simulink model "sampleModel344"  (R2021b)
settings: Solver=VariableStepAuto  StartTime=0.0  StopTime=10.0  RelTol=1e-3
undefined symbols (not defined in the file or in its folder): DiscIntNeverNeededParam
libraries: simulink x1
settings Model: Creator=user  LastModifiedBy=user

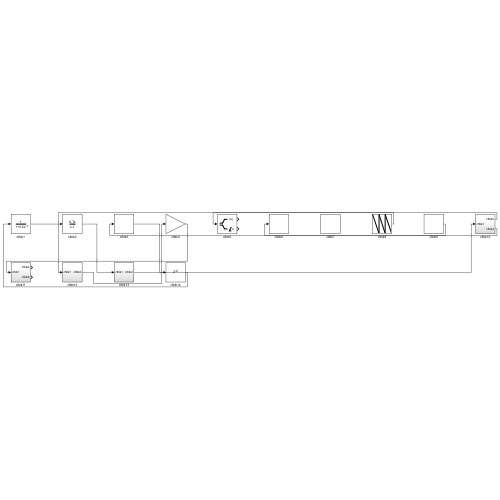
[thumbnail: Simulink's stored preview of the top-level diagram]
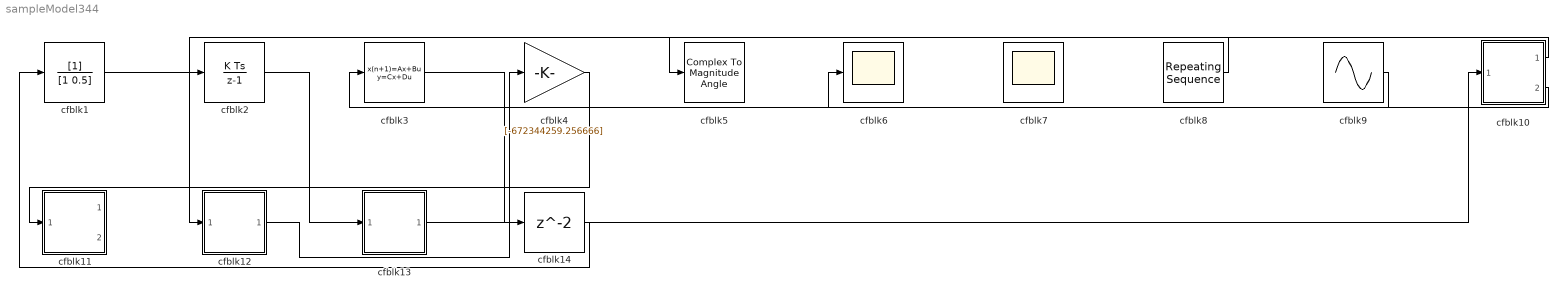
== system sampleModel344 ==
  cfblk1 : DiscreteFilter  SampleTime=1
  cfblk10 : Subsystem
  cfblk11 : Subsystem
  cfblk12 : Subsystem
  cfblk13 : Subsystem
  cfblk14 : Delay  SampleTime=1
  cfblk2 : DiscreteIntegrator  ICPrevOutput=DiscIntNeverNeededParam  ICPrevScaledInput=DiscIntNeverNeededParam
  cfblk3 : DiscreteStateSpace
  cfblk4 : Gain  Gain=[-672344259.256666]
  cfblk5 : ComplexToMagnitudeAngle
  cfblk6 : Scope
  cfblk7 : Scope
      settings: Floating=on
  cfblk8 : simulink/Sources/Repeating Sequence  rep_seq_t=[0 2]  rep_seq_y=[733938760.116119, 304654345.352208]
  cfblk9 : Sin  Amplitude=[225680626.132286]  Bias=[981324259.731864]  SampleTime=0
  wires:
  cfblk2/1 -> cfblk13/1(cfblk1)
  cfblk12/1(cfblk2) -> cfblk4/1
  cfblk10/1(cfblk2) -> cfblk12/1(cfblk1)
  cfblk9/1 -> cfblk6/1
  cfblk1/1 -> cfblk2/1
  cfblk8/1 -> cfblk5/1
  cfblk10/2(cfblk3) -> cfblk3/1
  cfblk13/1(cfblk2) -> cfblk10/1(cfblk1)
  cfblk4/1 -> cfblk11/1(cfblk1)
  cfblk3/1 -> cfblk14/1
  cfblk14/1 -> cfblk1/1

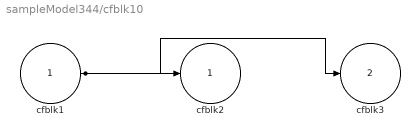
== system sampleModel344/cfblk10 ==
  cfblk1 : Inport
  cfblk2 : Outport
  cfblk3 : Outport  Port=2
  wires:
  cfblk1/1 -> cfblk2/1, cfblk3/1

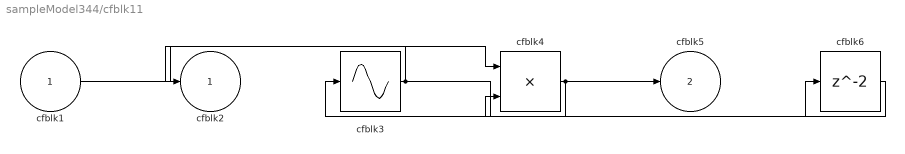
== system sampleModel344/cfblk11 ==
  cfblk1 : Inport
  cfblk3 : Sin  TimeSource=Use external signal  SampleTime=0
  cfblk4 : Product  Inputs=**
  cfblk6 : Delay  SampleTime=1
  cfblk2 : Outport
  cfblk5 : Outport  Port=2
  wires:
  cfblk1/1 -> cfblk4/1
  cfblk4/1 -> cfblk3/1, cfblk5/1
  cfblk3/1 -> cfblk2/1, cfblk6/1
  cfblk6/1 -> cfblk4/2

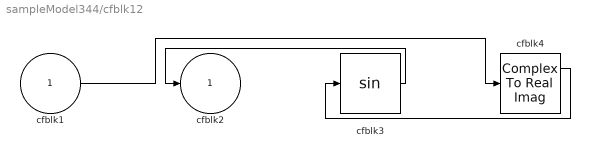
== system sampleModel344/cfblk12 ==
  cfblk1 : Inport
  cfblk3 : Trigonometry
  cfblk4 : ComplexToRealImag
  cfblk2 : Outport
  wires:
  cfblk3/1 -> cfblk2/1
  cfblk4/1 -> cfblk3/1
  cfblk1/1 -> cfblk4/1

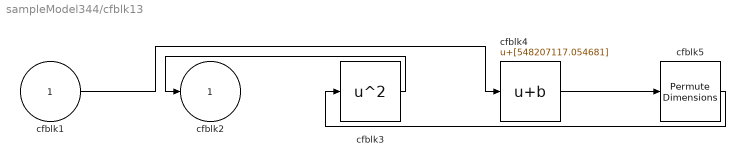
== system sampleModel344/cfblk13 ==
  cfblk1 : Inport
  cfblk3 : Math  Operator=square  SaturateOnIntegerOverflow=on
  cfblk4 : Bias  Bias=[548207117.054681]
  cfblk5 : PermuteDimensions
  cfblk2 : Outport
  wires:
  cfblk3/1 -> cfblk2/1
  cfblk5/1 -> cfblk3/1
  cfblk1/1 -> cfblk4/1
  cfblk4/1 -> cfblk5/1
